simulink model "dyanamic_Absorber_Model"  (R2020a)
settings: Solver=VariableStepAuto  StartTime=0.0  StopTime=10.0  RelTol=1e-3
undefined symbols (not defined in the file): b, F, K1, M1, M2, w0
settings Model: Creator=INDRAJIT MARATHE  LastModifiedBy=INDRAJIT MARATHE

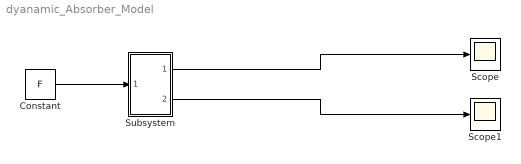
== system dyanamic_Absorber_Model ==
  Constant : Constant  Value=F
  Scope : Scope
  Scope1 : Scope
  Subsystem : Subsystem
  wires:
  Constant/1 -> Subsystem/1(In1)
  Subsystem/1(Output) -> Scope/1
  Subsystem/2(Output1) -> Scope1/1

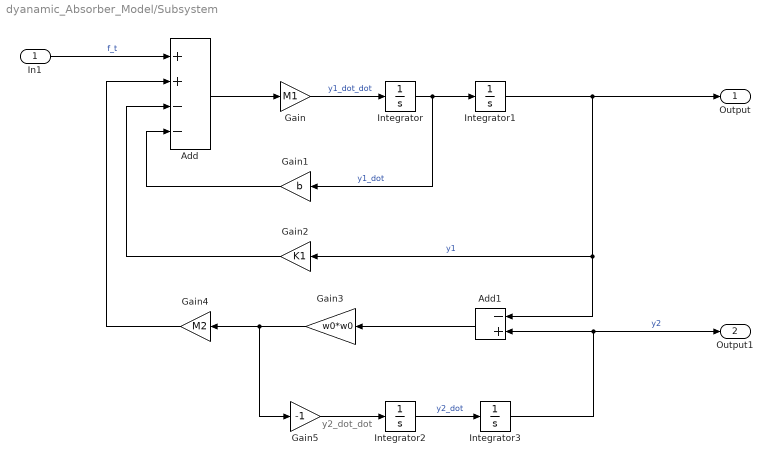
== system dyanamic_Absorber_Model/Subsystem ==
  note: y2_dot_dot
  In1 : Inport
  Add : Sum  Inputs=++--
  Add1 : Sum  Inputs=-+
  Gain : Gain  Gain=M1
  Gain1 : Gain  Gain=b
  Gain2 : Gain  Gain=K1
  Gain3 : Gain  Gain=w0*w0
  Gain4 : Gain  Gain=M2
  Gain5 : Gain  Gain=-1
  Integrator{,1..3} (4 alike) : Integrator
  Output : Outport
  Output1 : Outport  Port=2
  wires:
  Integrator2/1 -> Integrator3/1  "y2_dot"
  Integrator1/1 -> Output/1, Gain2/1, Add1/1  "y1"
  Gain1/1 -> Add/4
  Integrator/1 -> Integrator1/1, Gain1/1  "y1_dot"
  Add1/1 -> Gain3/1
  Gain5/1 -> Integrator2/1
  Integrator3/1 -> Output1/1, Add1/2  "y2"
  Gain2/1 -> Add/3
  Gain3/1 -> Gain5/1, Gain4/1
  Add/1 -> Gain/1
  Gain/1 -> Integrator/1  "y1_dot_dot"
  Gain4/1 -> Add/2
  In1/1 -> Add/1  "f_t"
